simulink model "Identify_model_right"  (R2015b)
settings: Solver=VariableStepAuto  StartTime=0.0  StopTime=147  RelTol=1e-3
values from neighbouring files (symbols this model uses):
  a0 = 0.0424941737179    [Identify_right.mat]
  a1 = 0.246207630573    [Identify_right.mat]
  b0 = 0.047154360386    [Identify_right.mat]
  r = 2.0276362585    [Identify_right.mat]
  sample_time = 1    [Identify_right.mat]
settings Model: Creator=ryodo  LastModifiedBy=ryodo

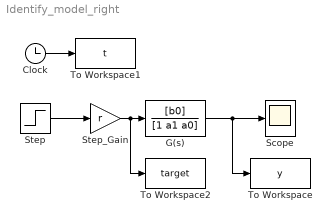
== system Identify_model_right ==
  Clock : Clock
  G(s) : TransferFcn  Numerator=[b0]  Denominator=[1 a1 a0]
  Scope : Scope
  Step : Step  Time=0  SampleTime=sample_time
  Step_Gain : Gain  Gain=r
  To Workspace : ToWorkspace  VariableName=y  SampleTime=sample_time
  To Workspace1 : ToWorkspace  VariableName=t  SampleTime=sample_time
  To Workspace2 : ToWorkspace  VariableName=target  SampleTime=sample_time
  wires:
  Step_Gain/1 -> To Workspace2/1, G(s)/1
  Step/1 -> Step_Gain/1
  G(s)/1 -> Scope/1, To Workspace/1
  Clock/1 -> To Workspace1/1
